simulink model "aoa_simulation"  (R2017b)
settings: Solver=FixedStepAuto  StartTime=0.0  StopTime=0.003  FixedStep=1e-8  RelTol=1e-3
InitFcn:
  | % Parameters of the system
  | f=2.421e9;    % Hz
  | D=0.0619;    % m
  | 
  | R=3;    % m
  | 
  | 
  | % Constants
  | c=physconst('LightSpeed');    % m/s
  | 
  | % Signal to noise ratio
  | SNR=20;
  | A_n=10^(-SNR/20);
undefined symbols (not defined in the file or in its folder): gaussian, jsin
libraries: simulink x2
settings Model: Creator=Antonio  LastModifiedBy=Antonio

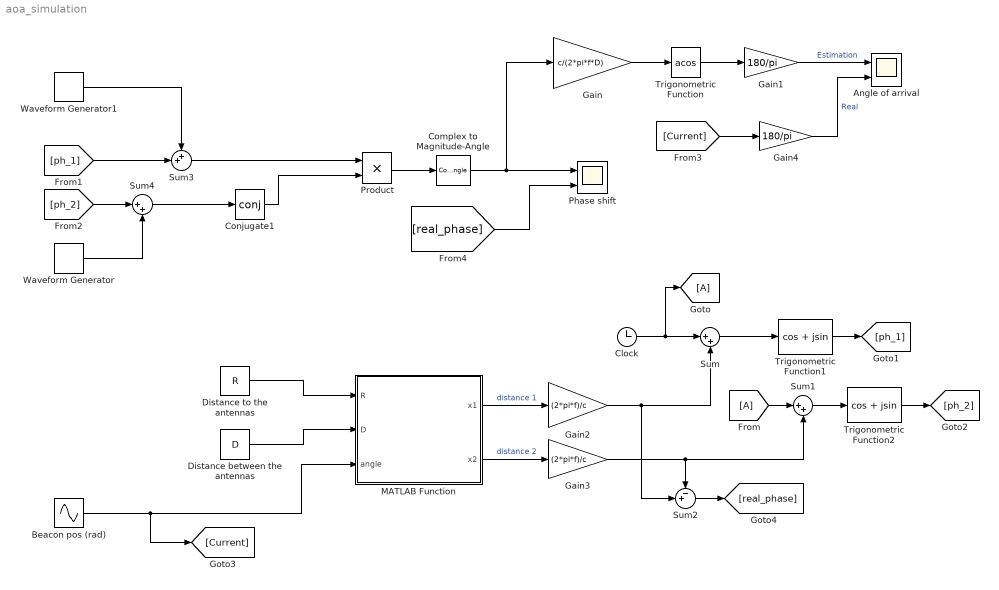
== system aoa_simulation ==
  "Angle of arrival " : Scope  NumInputPorts=2
  Beacon pos (rad) : Sin  Amplitude=pi  Frequency=2*pi*600  SampleTime=0
  Clock : Clock
  Complex to Magnitude-Angle : ComplexToMagnitudeAngle  Output=Angle
  Conjugate1 : Math  Operator=conj  RndMeth=Zero  SaturateOnIntegerOverflow=on
  Distance between the antennas : Constant  Value=D
  Distance to the antennas : Constant  Value=R
  Gain : Gain  Gain=c/(2*pi*f*D)
  Gain1 : Gain  Gain=180/pi
  Gain2 : Gain  Gain=(2*pi*f)/c
  Gain3 : Gain  Gain=(2*pi*f)/c
  Gain4 : Gain  Gain=180/pi
  MATLAB Function : MATLAB Function  TreatAsAtomicUnit=on
  Phase shift : Scope  NumInputPorts=2
  Product : Product
  Sum : Sum  Inputs=|++
  Sum1 : Sum  Inputs=|++
  Sum2 : Sum  Inputs=-+|
  Sum3 : Sum  Inputs=++|
  Sum4 : Sum  Inputs=|++
  Trigonometric Function : Trigonometry  Operator=acos  OutputSignalType=complex
  Trigonometric Function1 : Trigonometry  Operator=cos + jsin
  Trigonometric Function2 : Trigonometry  Operator=cos + jsin
  Waveform Generator : simulink/Sources/Waveform Generator  OutMin=[]  OutMax=[]  OutDataTypeStr=double  SelectedSignal=1  Signals=A_n*gaussian('Mean',0,'Variance',1,'Seed',354)  BlockNames=MultiportSwitch_667f555c30804d7  SampleTime=0.1
      settings: SourceProductName=Simulink
  Waveform Generator1 : simulink/Sources/Waveform Generator  OutMin=[]  OutMax=[]  OutDataTypeStr=double  SelectedSignal=1  Signals=A_n*gaussian('Mean',0,'Variance',1,'Seed',1)  BlockNames=MultiportSwitch_9de28b83f9ab491  SampleTime=0.1
      settings: SourceProductName=Simulink
  wires:
  Product/1 -> Complex to Magnitude-Angle/1
  Complex to Magnitude-Angle/1 -> Gain/1, Phase shift/1
  [real_phase] -> Phase shift/2
  Gain/1 -> Trigonometric Function/1
  Trigonometric Function/1 -> Gain1/1
  Gain1/1 -> "Angle of arrival "/1  "Estimation"
  Distance to the antennas/1 -> MATLAB Function/1(R)
  Distance between the antennas/1 -> MATLAB Function/2(D)
  MATLAB Function/2(x2) -> Gain3/1  "distance 2"
  MATLAB Function/1(x1) -> Gain2/1  "distance 1"
  Gain2/1 -> Sum/2, Sum2/2
  Clock/1 -> [A], Sum/1
  Gain3/1 -> Sum2/1, Sum1/2
  [A] -> Sum1/1
  Sum/1 -> Trigonometric Function1/1
  Sum1/1 -> Trigonometric Function2/1
  Trigonometric Function1/1 -> [ph_1]
  Trigonometric Function2/1 -> [ph_2]
  [Current] -> Gain4/1
  Gain4/1 -> "Angle of arrival "/2  "Real"
  Conjugate1/1 -> Product/2
  Sum2/1 -> [real_phase]
  Beacon pos (rad)/1 -> MATLAB Function/3(angle), [Current]
  Sum4/1 -> Conjugate1/1
  Waveform Generator/1 -> Sum4/2
  [ph_2] -> Sum4/1
  [ph_1] -> Sum3/2
  Sum3/1 -> Product/1
  Waveform Generator1/1 -> Sum3/1

== matlab function aoa_simulation/MATLAB Function ==
  data: R input; x1 output; D input; angle input; x2 output
function [x1, x2] = antenna_distances(R, D, angle)
%% This function computes the distances from the beacon
% to each antennas as a function of the following parameters
% R -> distance from the beacon to the middle point (m)
% D -> distance between the antennas (m)
% angle -> angle of the beacon with respect to the positive
% x-axis

%% Beacon distance and antenna positioning
x_A = R-D/2;                        % Antennas' position
x_B = R+D/2;

%% Compute angles of arrival to antennas
x_s = R*(1+cos(angle));             % Beacon's coordinates (4-quadrant)
y_s = R*abs(sin(angle-pi));
aoa_A = atan2(y_s, abs(x_s-x_A));   % Angles of arrival to both antennas (4-quadrant)
aoa_B = atan2(y_s, abs(x_s-x_B));

%% Compute distances from beacon to antennas
x1 = (abs(x_s-x_A))/cos(aoa_A);     % Distance of flight to antennas (4-quadrant)
x2 = (abs(x_s-x_B))/cos(aoa_B);
